simulink model "task3"  (Simulink 8.3)
settings: Solver=ode45  StartTime=0.0  StopTime=20.0  RelTol=1e-3
settings Model: Creator=Радион  LastModifiedBy=Радион
settings OptimizationCC: BooleanDataType=off
settings DebuggingCC: SaveWithParameterizedLinksMsg=none  SignalResolutionControl=TryResolveAllWithWarning  SolverPrmCheckMsg=none  MultiTaskDSMMsg=warning  MultiTaskCondExecSysMsg=none  StateNameClashWarn=none
settings HardwareCC: TargetUnknown=on
settings RTWCC: IncludeERTFirstTime=on

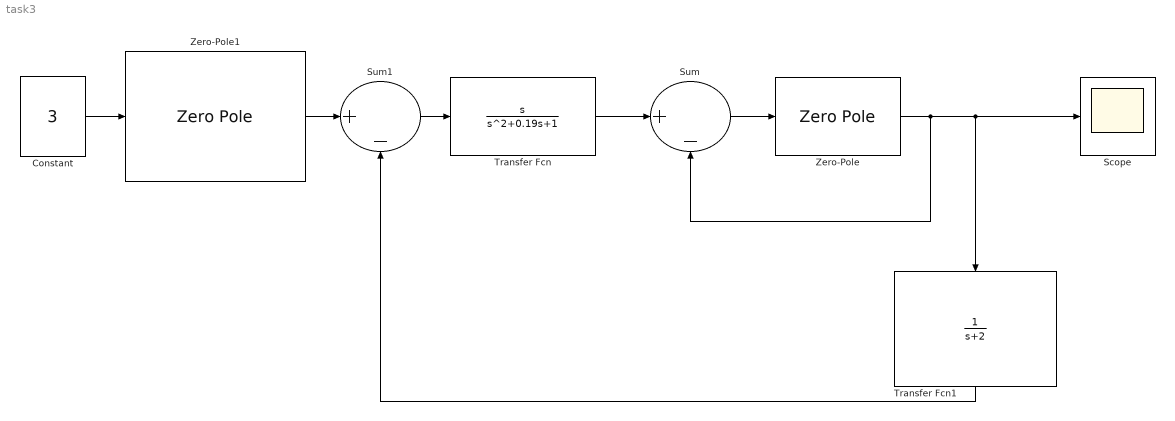
== system task3 ==
  Constant : Constant  Value=3
  Scope : Scope
      settings: TimeRange=10  YMin=-10000  YMax=10000
  Sum : Sum  Inputs=|+-  SaturateOnIntegerOverflow=on  InputSameDT=on  OutDataTypeStr=Inherit: Same as first input
  Sum1 : Sum  Inputs=|+-  SaturateOnIntegerOverflow=on  InputSameDT=on  OutDataTypeStr=Inherit: Same as first input
  Transfer Fcn : TransferFcn  Numerator=[1 0]  Denominator=[1 0.19 1]
  Transfer Fcn1 : TransferFcn  Denominator=[1 2]
  Zero-Pole : ZeroPole  Zeros=[0]  Poles=[-0.03 -1]
  Zero-Pole1 : ZeroPole  Zeros=[1 2 -1]  Poles="[0 -4  -3]"
  wires:
  Sum1/1 -> Transfer Fcn/1
  Transfer Fcn/1 -> Sum/1
  Sum/1 -> Zero-Pole/1
  Constant/1 -> Zero-Pole1/1
  Zero-Pole1/1 -> Sum1/1
  Zero-Pole/1 -> Sum/2, Scope/1, Transfer Fcn1/1
  Transfer Fcn1/1 -> Sum1/2
